simulink model "auto_vzmac_core"  (Simulink 7.9)
(part 3 of 4)

      | <!DOCTYPE HTML PUBLIC "-//W3C//DTD HTML 4.0//EN" "http://www.w3.org/TR/REC-html40/strict.dtd">
      | <html><head><meta name="qrichtext" content="1" /><style type="text/css">
      | p, li { white-space: pre-wrap; }
      | </style></head><body style=" font-family:'Sans'; font-size:10pt; font-weight:400; font-style:normal;">
      | <p style=" margin-top:0px; margin-bottom:0px; margin-left:0px; margin-right:0px; -qt-block-indent:0; text-indent:0px;"><img src="/tools/commercial/xilinx/14.6/ISE_DS/ISE/sysgen/data/images/xbip_dsp48_macro_v2_1_regimag.png" /></p></body></html>
      settings: infoedit=<html>Valid operands: CONCAT, P, C, PCIN, P>>17, PCIN>>17, CARRYIN, CARRYCASCIN, ACIN, A, BCIN,B<br><br>Valid operators: +, -, *, ()<br><br>Valid functions: RNDSIMPLE, RNDSYM<br><br>Instructions are case insensitive and tolerate spaces.</html>
  delay_bram : Subsystem  AncestorBlock=casper_library_delays/delay_bram  mask(delay_bram){DelayLen=2048-5, bram_latency=3, use_dsp48=on, async=off}
      mask prompts: DelayLen "Delay By:"; bram_latency "BRAM Latency"; use_dsp48 "Use DSP48"; async "asynchronous operation"
      mask help: A delay block that uses BRAM for its storage.
      mask init:
      | delay_bram_init(gcb, ...
      |     'DelayLen', DelayLen, ...
      |     'bram_latency', bram_latency, ...
      |     'use_dsp48', use_dsp48, ...
      |     'async', async);
      mask Help: eval('xlWeb(''http://casper.berkeley.edu/wiki/Delay_bram'')')
  valid : Outport
  re : Outport  Port=2
  wires:
  bd/2 -> ac/3
  ac/1 -> delay_bram/1(din)  "p"
  delay_bram/1(dout) -> Delay2/1, Assert/1  "prev"
  init/1 -> Delay1/1, Reinterpret/1
  Reinterpret/1 -> bd/4
  bd/1 -> Terminator/1
  Delay1/1 -> valid/1  "valid"
  a/1 -> ac/1
  Delay2/1 -> re/1  "re"
  c/1 -> ac/2
  b/1 -> bd/1
  d/1 -> bd/2
  Assert/1 -> bd/3
